simulink model "Logic112"  (R2016b)
settings: Solver=VariableStepAuto  StartTime=0.0  StopTime=10.0  RelTol=1e-3
libraries: simulink x1
settings Model: Creator=viett  LastModifiedBy=viett

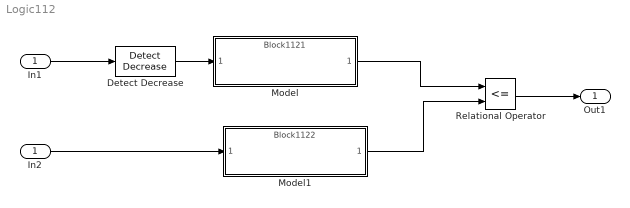
== system Logic112 ==
  In1 : Inport
  Detect Decrease : simulink/Logic and Bit Operations/Detect Decrease  vinit=0.0  OutDataTypeStr=boolean
  In2 : InportShadow
  Model : ModelReference  ModelNameDialog=Block1121.slx  SimulationMode=Normal  ModelReferenceVersion=1.1
  Model1 : ModelReference  ModelNameDialog=Block1122.slx  SimulationMode=Normal  ModelReferenceVersion=1.1
  Relational Operator : RelationalOperator  Operator=<=  OutDataTypeStr=boolean  RndMeth=Simplest
  Out1 : Outport
  wires:
  Model/1 -> Relational Operator/1
  Model1/1 -> Relational Operator/2
  Relational Operator/1 -> Out1/1
  Detect Decrease/1 -> Model/1
  In1/1 -> Detect Decrease/1
  In2/1 -> Model1/1
